simulink model "extra_robot_stuff"  (R2012b)
settings: Solver=ode45  StartTime=0.0  StopTime=10.0  RelTol=1e-3
settings Model: Creator=Dan  LastModifiedBy=Dan

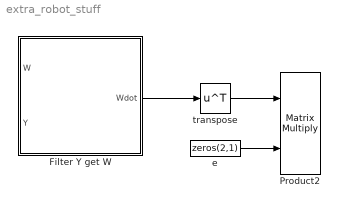
== system extra_robot_stuff ==
  Filter Y get W : MATLAB Function  TreatAsAtomicUnit=on
  Product2 : Product  Multiplication=Matrix(*)  RndMeth=Zero
  e : Constant  Value=zeros(2,1)
  transpose : Math  Operator=transpose  SaturateOnIntegerOverflow=on
  wires:
  transpose/1 -> Product2/1
  e/1 -> Product2/2
  Filter Y get W/1(Wdot) -> transpose/1

== matlab function extra_robot_stuff/Filter Y get W ==
  data: W input; Y input; Wdot output
%%%%%%%%%%%%%%%%%%%%%%%%%%%%%%%%%%%%%%%%%%%%%%%%%%%%%%%%%%%%%%%%%%%%%%%%%%%
% Daniel Wiese
% 2.152
% Robot Manipulator
%--------------------------------------------------------------------------
% Robot
%%%%%%%%%%%%%%%%%%%%%%%%%%%%%%%%%%%%%%%%%%%%%%%%%%%%%%%%%%%%%%%%%%%%%%%%%%%
function Wdot=fcn(W,Y)
%#codegen
%Preallocate output
Wdot=zeros(2,9);
lambdaf=100;
% %Take apart the input
% q1=q(1);
% q2=q(2);
% q_dot1=q_dot(1);
% q_dot2=q_dot(2);
% qr_dot1=qr_dot(1);
% qr_dot2=qr_dot(2);
% qr_ddot1=qr_ddot(1);
% qr_ddot2=qr_ddot(2);
% %Calculate the first row of Y
% Y(1,1)=qr_ddot1;
% Y(1,2)=qr_ddot2;
% Y(1,3)=(2*qr_ddot1+qr_ddot2)*cos(q2)-(q_dot2*qr_dot1+q_dot1*qr_dot2+q_dot2*qr_dot2)*sin(q2);
% Y(1,4)=(2*qr_ddot1+qr_ddot2)*sin(q2)+(q_dot2*qr_dot1+q_dot1*qr_dot2+q_dot2*qr_dot2)*cos(q2);
% Y(1,5)=cos(q1);
% Y(1,6)=cos(q1+q2);
% Y(1,7)=-sin(q1+q2);
% Y(1,8)=q_dot1;
% Y(1,9)=0;
% %Calculate the second row of Y
% Y(2,1)=0;
% Y(2,2)=qr_ddot1+qr_ddot2;
% Y(2,3)=qr_ddot1*cos(q2)+q_dot1*qr_dot1*sin(q2);
% Y(2,4)=qr_ddot1*sin(q2)-q_dot1*qr_dot1*cos(q2);
% Y(2,5)=0;
% Y(2,6)=cos(q1+q2);
% Y(2,7)=-sin(q1+q2);
% Y(2,8)=0;
% Y(2,9)=q_dot2;

% Wdot=-lambdaf*W+lambdaf*Y;
